simulink model "p5_2015"  (R2015a)
settings: Solver=ode45  StartTime=0.0  StopTime=10.0  RelTol=1e-3
settings Model: Creator=sala3  LastModifiedBy=Sala3

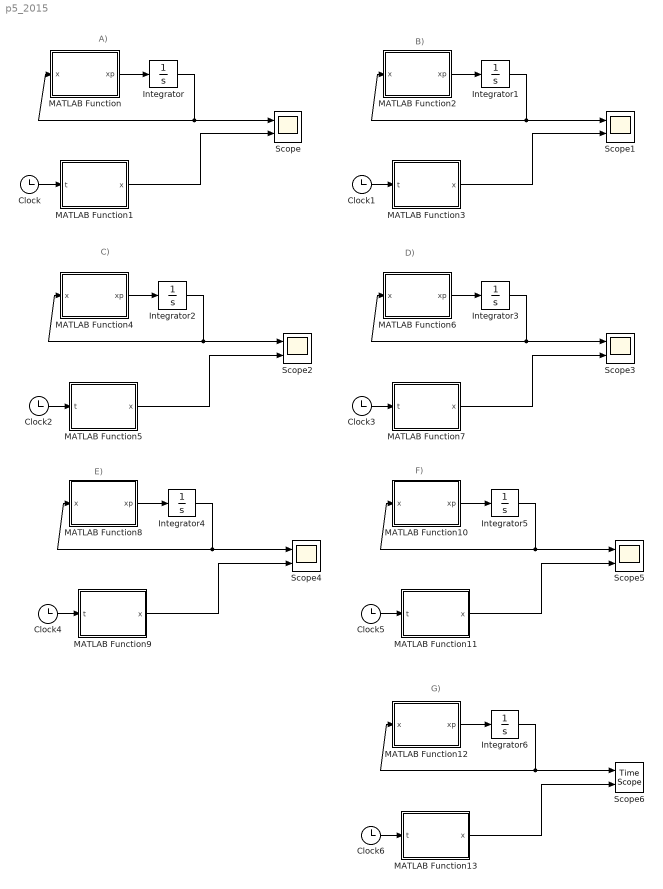
== system p5_2015 ==
  note: G)
  note: F)
  note: E)
  note: D)
  note: C)
  note: B)
  note: A)
  Clock{,1..6} (7 alike) : Clock
  Integrator : Integrator  InitialCondition=[2 3]
  Integrator1 : Integrator  InitialCondition=[4 3]
  Integrator2 : Integrator  InitialCondition=[2 4]
  Integrator3 : Integrator  InitialCondition=[5 4]
  Integrator4 : Integrator  InitialCondition=[5 3]
  Integrator5 : Integrator  InitialCondition=[4 6 3]
  Integrator6 : Integrator  InitialCondition=[5 4 3]
  MATLAB Function : MATLAB Function  TreatAsAtomicUnit=on
  MATLAB Function1 : MATLAB Function  TreatAsAtomicUnit=on
  MATLAB Function10 : MATLAB Function  TreatAsAtomicUnit=on
  MATLAB Function11 : MATLAB Function  TreatAsAtomicUnit=on
  MATLAB Function12 : MATLAB Function  TreatAsAtomicUnit=on
  MATLAB Function13 : MATLAB Function  TreatAsAtomicUnit=on
  MATLAB Function2 : MATLAB Function  TreatAsAtomicUnit=on
  MATLAB Function3 : MATLAB Function  TreatAsAtomicUnit=on
  MATLAB Function4 : MATLAB Function  TreatAsAtomicUnit=on
  MATLAB Function5 : MATLAB Function  TreatAsAtomicUnit=on
  MATLAB Function6 : MATLAB Function  TreatAsAtomicUnit=on
  MATLAB Function7 : MATLAB Function  TreatAsAtomicUnit=on
  MATLAB Function8 : MATLAB Function  TreatAsAtomicUnit=on
  MATLAB Function9 : MATLAB Function  TreatAsAtomicUnit=on
  Scope{,1..5} (6 alike) : Scope  NumInputPorts=2
      Scope settings: YMin=-2752.18477~-2752.18313  YMax=24779.66383~24779.64906
      Scope1 settings: YMin=-3.51912~-5  YMax=5.21202~5
      Scope2 settings: YMin=-0.5~-5  YMax=4.5~5  SaveName=ScopeData2
      Scope3 settings: YMin=-0.625~-5  YMax=5.625~5  SaveName=ScopeData3
      Scope4 settings: YMin=-23.74756~-23.74756  YMax=13.74756~13.74756  SaveName=ScopeData4
      Scope5 settings: YMin=-0.75~-5  YMax=6.75~5  SaveName=ScopeData5
  Scope6 : TimeScope  NumInputPorts=2
  wires:
  MATLAB Function/1(xp) -> Integrator/1
  Clock/1 -> MATLAB Function1/1(t)
  Integrator/1 -> Scope/1, MATLAB Function/1(x)
  MATLAB Function1/1(x) -> Scope/2
  MATLAB Function3/1(x) -> Scope1/2
  Integrator1/1 -> MATLAB Function2/1(x), Scope1/1
  Clock1/1 -> MATLAB Function3/1(t)
  MATLAB Function2/1(xp) -> Integrator1/1
  MATLAB Function5/1(x) -> Scope2/2
  Integrator2/1 -> MATLAB Function4/1(x), Scope2/1
  Clock2/1 -> MATLAB Function5/1(t)
  MATLAB Function4/1(xp) -> Integrator2/1
  MATLAB Function6/1(xp) -> Integrator3/1
  Clock3/1 -> MATLAB Function7/1(t)
  Integrator3/1 -> Scope3/1, MATLAB Function6/1(x)
  MATLAB Function7/1(x) -> Scope3/2
  MATLAB Function11/1(x) -> Scope5/2
  Integrator5/1 -> MATLAB Function10/1(x), Scope5/1
  Clock5/1 -> MATLAB Function11/1(t)
  MATLAB Function10/1(xp) -> Integrator5/1
  MATLAB Function8/1(xp) -> Integrator4/1
  Clock4/1 -> MATLAB Function9/1(t)
  Integrator4/1 -> Scope4/1, MATLAB Function8/1(x)
  MATLAB Function9/1(x) -> Scope4/2
  MATLAB Function12/1(xp) -> Integrator6/1
  Clock6/1 -> MATLAB Function13/1(t)
  Integrator6/1 -> Scope6/1, MATLAB Function12/1(x)
  MATLAB Function13/1(x) -> Scope6/2

== matlab function p5_2015/MATLAB Function1 ==
  data: x output; t input
function x = fcn(t)
%#codegen
x=[(3*exp(-t))/2 + exp(t)/2 + sinh(t);2*exp(-t) + 1];

== matlab function p5_2015/MATLAB Function ==
  data: x input; xp output
function xp = fcn(x)
%#codegen
u=1;
A=[1 -1;0 -1];
B=[1 1]';
xp=A*x+B*u;

== matlab function p5_2015/MATLAB Function2 ==
  data: x input; xp output
function xp = fcn(x)
%#codegen
A=[0 1;-4 -5];
B=[1 2]';
u=1;
xp=A*x+B*u;

== matlab function p5_2015/MATLAB Function3 ==
  data: x output; t input
function x = fcn(t)
%#codegen
x=[(13*exp(-t))/3 - (25*exp(-4*t))/12 + 7/4;(25*exp(-4*t))/3 - (13*exp(-t))/3 - 1];

== matlab function p5_2015/MATLAB Function4 ==
  data: x input; xp output
function xp = fcn(x)
%#codegen
A=[-3 1;0 -3];
B=[1 0]';
u=10;
xp=A*x+B*u;

== matlab function p5_2015/MATLAB Function5 ==
  data: x output; t input
function x = fcn(t)
%#codegen
x=[4*t*exp(-3*t) - (4*exp(-3*t))/3 + 10/3; 4*exp(-3*t)];

== matlab function p5_2015/MATLAB Function6 ==
  data: x input; xp output
function xp = fcn(x)
%#codegen
A=[-4 0;0 -3];
B=[0 1]';
u=5;
xp=A*x+B*u;

== matlab function p5_2015/MATLAB Function7 ==
  data: x output; t input
function x = fcn(t)
%#codegen
x=[5*exp(-4*t); (7*exp(-3*t))/3 + 5/3];

== matlab function p5_2015/MATLAB Function10 ==
  data: x input; xp output
function xp = fcn(x)
%#codegen
A=[-1 0 0;0 -2 1;0 0 -2];
B=[1 1 0]';
u=1;
xp=A*x+B*u;

== matlab function p5_2015/MATLAB Function11 ==
  data: x output; t input
function x = fcn(t)
%#codegen
x=[3*exp(-t) + 1; (11*exp(-2*t))/2 + 3*t*exp(-2*t) + 1/2;3*exp(-2*t)];

== matlab function p5_2015/MATLAB Function8 ==
  data: x input; xp output
function xp = fcn(x)
%#codegen
A=[0 1;-2 -3];
B=[1 1]';
u=-10;
xp=A*x+B*u;

== matlab function p5_2015/MATLAB Function9 ==
  data: x output; t input
function x = fcn(t)
%#codegen
x=[ 43*exp(-t) - 18*exp(-2*t) - 20;36*exp(-2*t) - 43*exp(-t) + 10];

== matlab function p5_2015/MATLAB Function12 ==
  data: x input; xp output
function xp = fcn(x)
%#codegen
A=[-5 1 0;0 -5 1;0 0 -5];
B=[1 0 1]';
u=1;
xp=A*x+B*u;

== matlab function p5_2015/MATLAB Function13 ==
  data: x output; t input
function x = fcn(t)
%#codegen
x=[(24*exp(-5*t))/5 + 4*t*exp(-5*t) + (3*t^2*exp(-5*t))/2 - (exp(-5*t)*(t^2/5 + (2*t)/25 + 2/125))/2 + 26/125;(99*exp(-5*t))/25 + (14*t*exp(-5*t))/5 + 1/25;(14*exp(-5*t))/5 + 1/5];
